simulink model "BehQCStation"  (R2026a)
settings: Solver=VariableStepAuto
model workspace (MAT data in the model file):
  CalibPeriod_s = 3600
  CalibTime_s = 60
  ContamIncidence = 0
  DetectSensitivity = 0.995
  QCRate_bph = 200
  RejectFrac = 0.02
settings Model: DataDictionary=BehParamsCommon.sldd  ParameterArgumentNames=QCRate_bph,RejectFrac,CalibPeriod_s,CalibTime_s,ContamIncidence,DetectSensitivity  Creator=sarah  LastModifiedBy=sarah

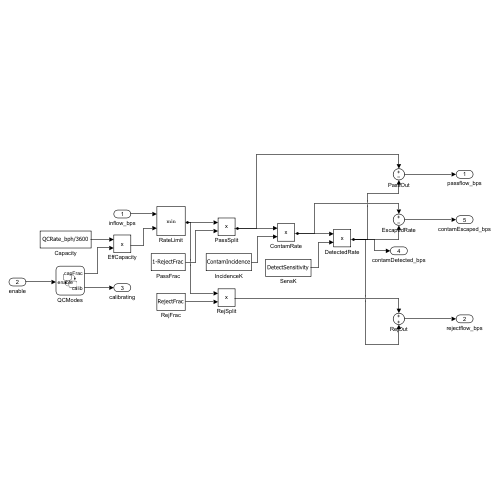
[thumbnail: Simulink's stored preview of the top-level diagram]
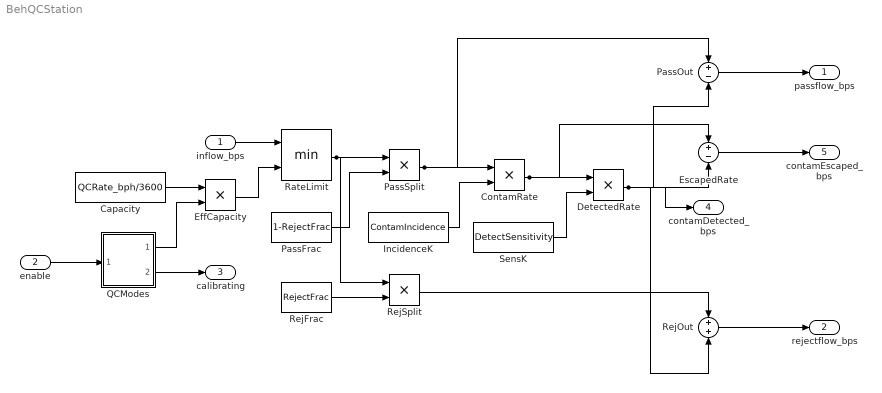
== system BehQCStation ==
  inflow_bps : Inport
  enable : Inport  Port=2
  Capacity : Constant  Value=QCRate_bph/3600
  ContamRate : Product
  DetectedRate : Product
  EffCapacity : Product
  EscapedRate : Sum  Inputs=+-
  IncidenceK : Constant  Value=ContamIncidence
  PassFrac : Constant  Value=1-RejectFrac
  PassOut : Sum  Inputs=+-
  PassSplit : Product
  QCModes : Stateflow chart  TreatAsAtomicUnit=on
  RateLimit : MinMax  Inputs=2
  RejFrac : Constant  Value=RejectFrac
  RejOut : Sum
  RejSplit : Product
  SensK : Constant  Value=DetectSensitivity
  passflow_bps : Outport
  rejectflow_bps : Outport  Port=2
  calibrating : Outport  Port=3
  contamDetected_bps : Outport  Port=4
  contamEscaped_bps : Outport  Port=5
  wires:
  enable/1 -> QCModes/1(enable)
  Capacity/1 -> EffCapacity/1
  QCModes/1(capFrac) -> EffCapacity/2
  RateLimit/1 -> RejSplit/1, PassSplit/1
  QCModes/2(calib) -> calibrating/1
  inflow_bps/1 -> RateLimit/1
  ContamRate/1 -> EscapedRate/1, DetectedRate/1
  PassFrac/1 -> PassSplit/2
  EffCapacity/1 -> RateLimit/2
  RejFrac/1 -> RejSplit/2
  PassSplit/1 -> PassOut/1, ContamRate/1
  IncidenceK/1 -> ContamRate/2
  RejSplit/1 -> RejOut/1
  SensK/1 -> DetectedRate/2
  DetectedRate/1 -> PassOut/2, contamDetected_bps/1, EscapedRate/2, RejOut/2
  PassOut/1 -> passflow_bps/1
  EscapedRate/1 -> contamEscaped_bps/1
  RejOut/1 -> rejectflow_bps/1

== stateflow chart BehQCStation/QCModes ==
  settings: updateMethod=DISCRETE  sampleTime=1
  state Inspecting
    du: capFrac = 1; calib = 0;
  state Calibrating
    du: capFrac = 0; calib = 1;
  state Disabled
    du: capFrac = 0; calib = 0;
  (default) -> Inspecting
  Calibrating -> Inspecting : [after(CalibTime_s, sec)]
  Inspecting -> Calibrating [order 2] : [after(CalibPeriod_s, sec)]
  Disabled -> Inspecting : [enable >= 0.5]
  Inspecting -> Disabled [order 1] : [enable < 0.5]
  data: enable input double; capFrac output double; calib output double; CalibPeriod_s parameter double; CalibTime_s parameter double
